simulink model "Simulazione_fisica"  (R2025b)
settings: Solver=ode15s  StartTime=0.0  StopTime=1  MaxStep=1e-2  RelTol=1e-6
InitFcn:
  | run("init.m");
undefined symbols (not defined in the file or in its folder): q1_init, q2_init
settings Model: Creator=Acer  LastModifiedBy=Acer
settings SolverCC: InitialStep=1e-5  SolverResetMethod=Robust

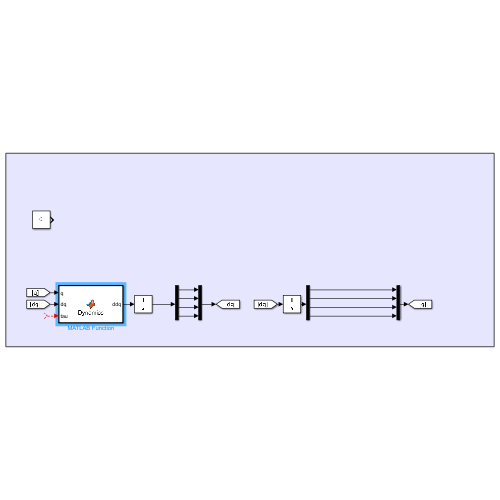
[thumbnail: Simulink's stored preview of the top-level diagram]
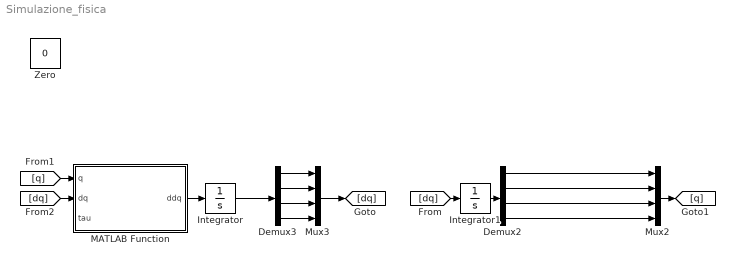
== system Simulazione_fisica ==
  Demux2 : Demux
  Demux3 : Demux
  Integrator : Integrator  InitialCondition=[0;0;0]  ContinuousStateAttributes="\"dq\""
  Integrator1 : Integrator  InitialCondition=[q1_init;0;q2_init]  ContinuousStateAttributes="\"q\""
  MATLAB Function : MATLAB Function  TreatAsAtomicUnit=on
  Mux2 : Mux
  Mux3 : Mux
  Zero : Constant  Value=0  OutDataTypeStr=Inherit: Inherit via back propagation
  wires:
  MATLAB Function/1(ddq) -> Integrator/1
  [dq] -> Integrator1/1
  [q] -> MATLAB Function/1(q)
  [dq] -> MATLAB Function/2(dq)
  Integrator1/1 -> Demux2/1
  Mux2/1 -> [q]
  Mux3/1 -> [dq]
  Integrator/1 -> Demux3/1
  ? -> MATLAB Function/3(tau)
  Demux3/2 -> Mux3/2
  Demux2/2 -> Mux2/2
  Demux2/1 -> Mux2/1
  Demux3/1 -> Mux3/1
  Demux3/3 -> Mux3/3
  Demux2/3 -> Mux2/3
  Demux3/4 -> Mux3/4
  Demux2/4 -> Mux2/4

== matlab function Simulazione_fisica/MATLAB Function ==
  settings: updateMethod=CONTINUOUS
  data: q input double size=3; dq input double size=3; tau input size=3; ddq output double size=3; robot_params parameter
function ddq = Dynamics(q,dq,tau,robot_params)


q1 = q(1);
qw = q(2);
q2 = q(3);
dq1 = dq(1);
dqw = dq(2);
dq2 = dq(3);

m1 = robot_params.m1;
m2 = robot_params.m2;
meq = robot_params.meq;
lc2 = robot_params.lc1;
lc1 = robot_params.lc2;
l1 = robot_params.l1;
l2 = robot_params.l2;
mw = robot_params.mw;
Rw = robot_params.Rw;
Iw= robot_params.Iw;
g = robot_params.g;
bw =  robot_params.bw;
b1 =  robot_params.b1;
b2 = robot_params.b2;
I1 = robot_params.I1;  
I2 = robot_params.I2;


[M,C,G] = 
 


ddq = M\(-C-G);
